simulink model "Magnetic_torque"  (R2021b)
settings: Solver=VariableStepAuto  StartTime=0.0  StopTime=10.0  RelTol=1e-3
libraries: matrix_library x2, simulink_extras x1, vrlib x1
settings Model: Creator=adity  LastModifiedBy=adity

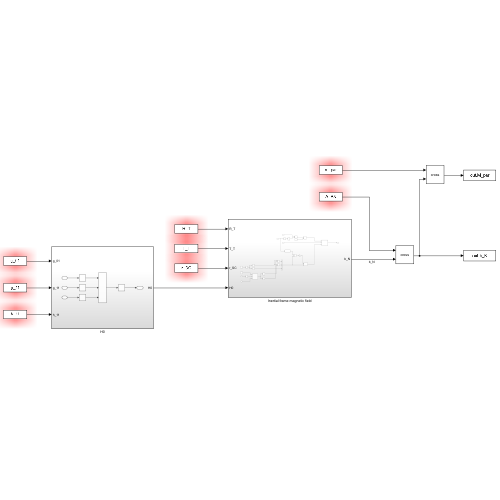
[thumbnail: Simulink's stored preview of the top-level diagram]
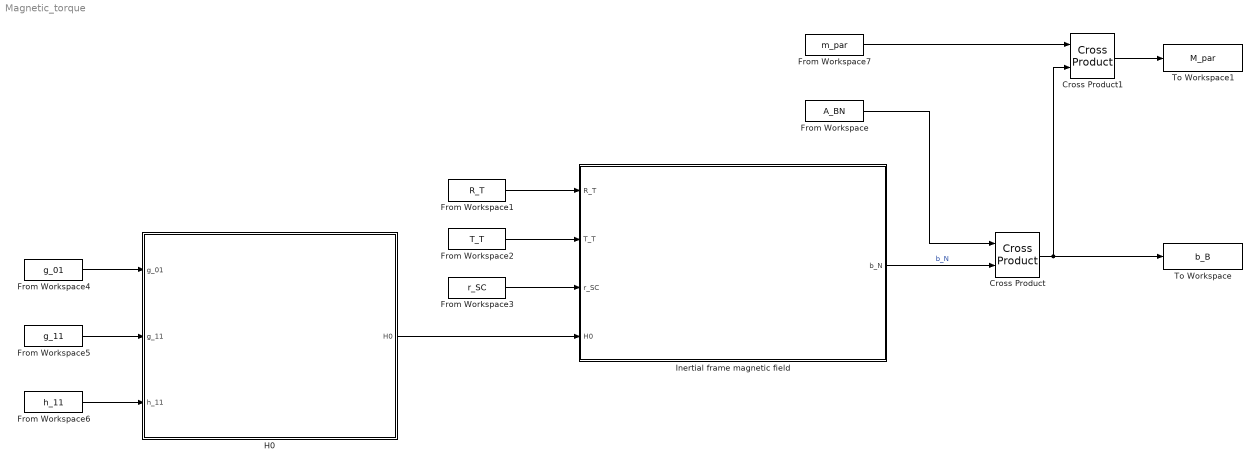
== system Magnetic_torque ==
  Cross Product : matrix_library/Cross Product
      settings: SourceProductBaseCode=SL
  Cross Product1 : matrix_library/Cross Product
      settings: SourceProductBaseCode=SL
  From Workspace : FromWorkspace  VariableName=A_BN
  From Workspace1 : FromWorkspace  VariableName=R_T
  From Workspace2 : FromWorkspace  VariableName=T_T
  From Workspace3 : FromWorkspace  VariableName=r_SC
  From Workspace4 : FromWorkspace  VariableName=g_01
  From Workspace5 : FromWorkspace  VariableName=g_11
  From Workspace6 : FromWorkspace  VariableName=h_11
  From Workspace7 : FromWorkspace  VariableName=m_par
  H0 : Subsystem
  Inertial frame magnetic field : Subsystem
  To Workspace : ToWorkspace  VariableName=b_B  SaveFormat=Timeseries  SampleTime=-1
  To Workspace1 : ToWorkspace  VariableName=M_par  SaveFormat=Timeseries  SampleTime=-1
  wires:
  From Workspace/1 -> Cross Product/1
  Inertial frame magnetic field/1(b_N) -> Cross Product/2  "b_N"
  From Workspace1/1 -> Inertial frame magnetic field/1(R_T)
  From Workspace2/1 -> Inertial frame magnetic field/2(T_T)
  From Workspace3/1 -> Inertial frame magnetic field/3(r_SC)
  H0/1(H0) -> Inertial frame magnetic field/4(H0)
  From Workspace6/1 -> H0/3(h_11)
  From Workspace5/1 -> H0/2(g_11)
  From Workspace4/1 -> H0/1(g_01)
  Cross Product/1 -> To Workspace/1, Cross Product1/2
  From Workspace7/1 -> Cross Product1/1
  Cross Product1/1 -> To Workspace1/1

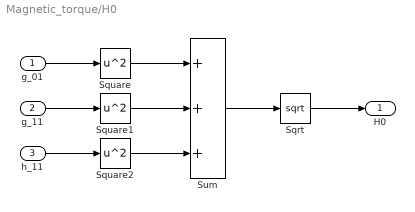
== system Magnetic_torque/H0 ==
  g_01 : Inport
  g_11 : Inport  Port=2
  h_11 : Inport  Port=3
  Sqrt : Sqrt  SaturateOnIntegerOverflow=on
  Square : Math  Operator=square  SaturateOnIntegerOverflow=on
  Square1 : Math  Operator=square  SaturateOnIntegerOverflow=on
  Square2 : Math  Operator=square  SaturateOnIntegerOverflow=on
  Sum : Sum  Inputs=+++
  H0 : Outport
  wires:
  Sqrt/1 -> H0/1
  Sum/1 -> Sqrt/1
  g_01/1 -> Square/1
  Square/1 -> Sum/1
  g_11/1 -> Square1/1
  Square1/1 -> Sum/2
  h_11/1 -> Square2/1
  Square2/1 -> Sum/3

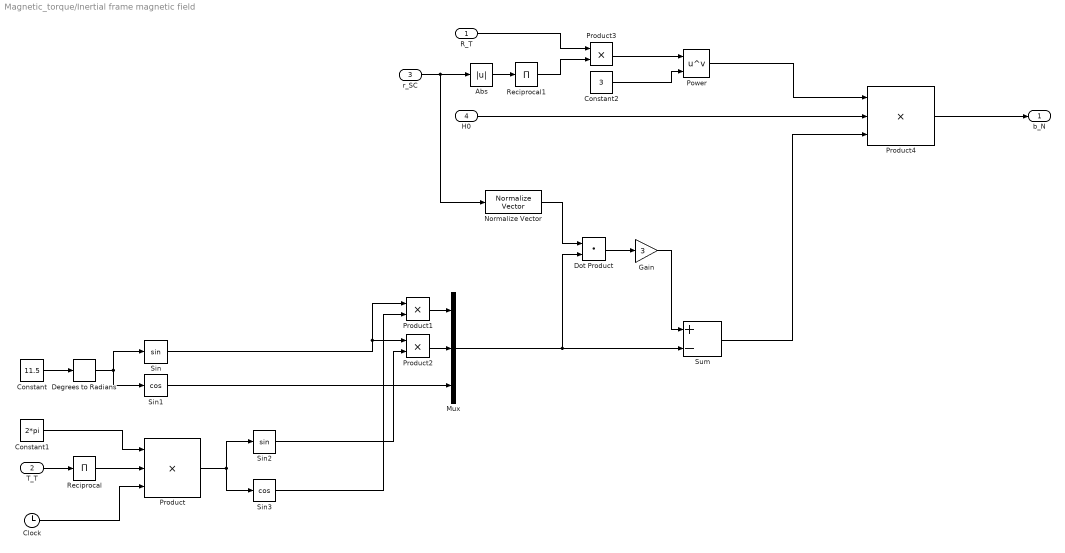
== system Magnetic_torque/Inertial frame magnetic field ==
  R_T : Inport
  T_T : Inport  Port=2
  r_SC : Inport  Port=3
  H0 : Inport  Port=4
  Abs : Abs
  Clock : Clock
  Constant : Constant  Value=11.5
  Constant1 : Constant  Value=2*pi
  Constant2 : Constant  Value=3
  Degrees to Radians : simulink_extras/Transformations/Degrees to Radians
  Dot Product : DotProduct  InputSameDT=on  OutDataTypeStr=Inherit: Inherit via internal rule
  Gain : Gain  Gain=3
  Mux : Mux  Inputs=3
  Normalize Vector : vrlib/Utilities/Normalize Vector  maxzero=0
  Power : Math  Operator=pow  SaturateOnIntegerOverflow=on
  Product : Product  Inputs=3
  Product1 : Product
  Product2 : Product
  Product3 : Product
  Product4 : Product  Inputs=3
  Reciprocal : Product  Inputs=1
  Reciprocal1 : Product  Inputs=1
  Sin : Trigonometry
  Sin1 : Trigonometry  Operator=cos
  Sin2 : Trigonometry
  Sin3 : Trigonometry  Operator=cos
  Sum : Sum  Inputs=+-
  b_N : Outport
  wires:
  Constant/1 -> Degrees to Radians/1
  Degrees to Radians/1 -> Sin1/1, Sin/1
  T_T/1 -> Reciprocal/1
  Reciprocal/1 -> Product/2
  Constant1/1 -> Product/1
  Clock/1 -> Product/3
  Product2/1 -> Mux/2
  Product1/1 -> Mux/1
  Sin1/1 -> Mux/3
  Product/1 -> Sin2/1, Sin3/1
  Sin/1 -> Product1/1, Product2/1
  Sin3/1 -> Product1/2
  Sin2/1 -> Product2/2
  r_SC/1 -> Abs/1, Normalize Vector/1
  R_T/1 -> Product3/1
  Reciprocal1/1 -> Product3/2
  Product3/1 -> Power/1
  Constant2/1 -> Power/2
  H0/1 -> Product4/2
  Power/1 -> Product4/1
  Abs/1 -> Reciprocal1/1
  Normalize Vector/1 -> Dot Product/1
  Mux/1 -> Dot Product/2, Sum/2
  Dot Product/1 -> Gain/1
  Gain/1 -> Sum/1
  Sum/1 -> Product4/3
  Product4/1 -> b_N/1
